simulink model "beachball"  (R2022b)
settings: Solver=VariableStepAuto  StartTime=0.0  StopTime=10.0  RelTol=1e-3
libraries: VACLib x7
settings Model: Creator=KarlO  LastModifiedBy=KarlO

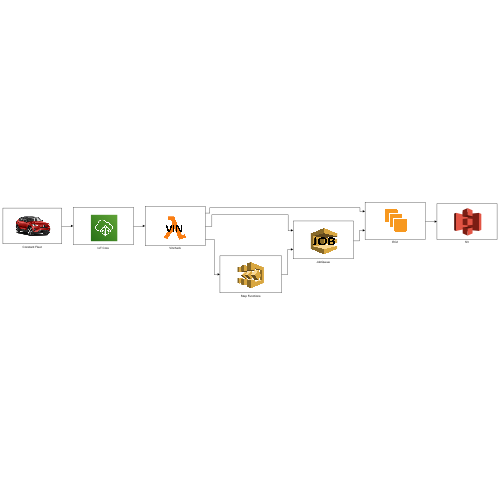
[thumbnail: Simulink's stored preview of the top-level diagram]
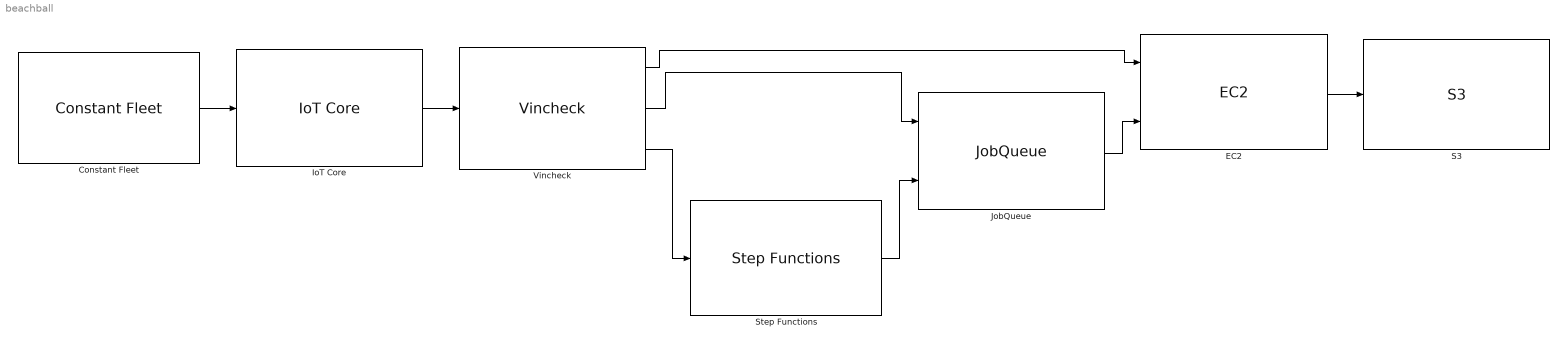
== system beachball ==
  Constant Fleet : VACLib/Vehicle Components/Constant Fleet  SystemSampleTime=-1  VariantActivationTime=update diagram  Latency=0  AutoFrameSizeCalculation=off
      settings: SourceProductName=Volvo Architechture Components
  EC2 : VACLib/AWS Components/EC2  SystemSampleTime=-1  VariantActivationTime=update diagram  Latency=0  AutoFrameSizeCalculation=off
      settings: SourceProductName=Volvo Architechture Components
  IoT Core : VACLib/AWS Components/IoT Core  SystemSampleTime=-1  VariantActivationTime=update diagram  Latency=0  AutoFrameSizeCalculation=off
      settings: SourceProductName=Volvo Architechture Components
  JobQueue : VACLib/AWS Components/JobQueue  SystemSampleTime=-1  VariantActivationTime=update diagram  Latency=0  AutoFrameSizeCalculation=off
      settings: SourceProductName=Volvo Architechture Components
  S3 : VACLib/AWS Components/S3  SystemSampleTime=-1  VariantActivationTime=update diagram  Latency=0  AutoFrameSizeCalculation=off
      settings: SourceProductName=Volvo Architechture Components
  Step Functions : VACLib/AWS Components/Step Functions  SystemSampleTime=-1  VariantActivationTime=update diagram  Latency=0  AutoFrameSizeCalculation=off
      settings: SourceProductName=Volvo Architechture Components
  Vincheck : VACLib/AWS Components/Vincheck  SystemSampleTime=-1  VariantActivationTime=update diagram  Latency=0  AutoFrameSizeCalculation=off
      settings: SourceProductName=Volvo Architechture Components
  wires:
  Constant Fleet/1 -> IoT Core/1
  IoT Core/1 -> Vincheck/1
  Step Functions/1 -> JobQueue/2
  Vincheck/1 -> EC2/1
  EC2/1 -> S3/1
  Vincheck/2 -> JobQueue/1
  Vincheck/3 -> Step Functions/1
  JobQueue/1 -> EC2/2
